simulink model "zerocross"  (Simulink 4.00)
settings: Solver=ode45  StartTime=0.0  StopTime=10.0  RelTol=1e-3
settings Model: LastModifiedBy=dev  LimitDataPoints=off  RTWOptions="-aExtMode=0 -aForceParamTrailComments=0 -aInlineInvariantSignals=0 -aLocalBlockOutputs=1 -aLogVarNameModifier=\"rt_\" -aRTWVerbose=1 -aRollThreshold=5 -aShowEliminatedStatements=1"  RTWInlineParameters=on  BlockReductionOpt=off

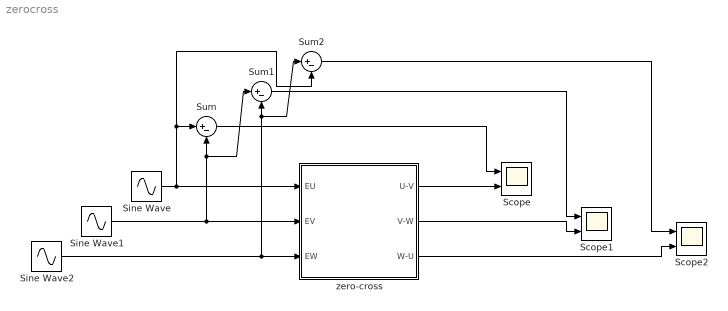
== system zerocross ==
  Scope : Scope  NumInputPorts=2
      settings: TimeRange=auto  YMin=-5~-5  YMax=5~5  SaveToWorkspace=off  SaveName=ScopeData  MaxDataPoints=5000
  Scope1 : Scope  NumInputPorts=2
      settings: TimeRange=auto  YMin=-5~-5  YMax=5~5  SaveToWorkspace=off  MaxDataPoints=5000
  Scope2 : Scope  NumInputPorts=2
      settings: TimeRange=auto  YMin=-5~-5  YMax=5~5  SaveToWorkspace=off  SaveName=ScopeData2  MaxDataPoints=5000
  Sine Wave : Sin  Amplitude=1  Frequency=10  Phase=0  SampleTime=0
  Sine Wave1 : Sin  Amplitude=1  Frequency=10  Phase=2*pi/3  SampleTime=0
  Sine Wave2 : Sin  Amplitude=1  Frequency=10  Phase=-2*pi/3  SampleTime=0
  Sum : Sum  Inputs=|+-  SaturateOnIntegerOverflow=on
  Sum1 : Sum  Inputs=|+-  SaturateOnIntegerOverflow=on
  Sum2 : Sum  Inputs=|+-  SaturateOnIntegerOverflow=on
  zero-cross : Subsystem
      settings: RTWFcnNameOpts=Auto  RTWFileNameOpts=Auto
      mask Description: The block detects the zero crossing of the inputs. For accurate results use the  rising edge only.
  wires:
  Sine Wave/1 -> zero-cross/1(EU), Sum/1, Sum2/2
  Sine Wave1/1 -> zero-cross/2(EV), Sum/2, Sum1/1
  Sine Wave2/1 -> zero-cross/3(EW), Sum1/2, Sum2/1
  zero-cross/1(U-V) -> Scope/2
  Sum/1 -> Scope/1
  Sum1/1 -> Scope1/1
  zero-cross/2(V-W) -> Scope1/2
  Sum2/1 -> Scope2/1
  zero-cross/3(W-U) -> Scope2/2

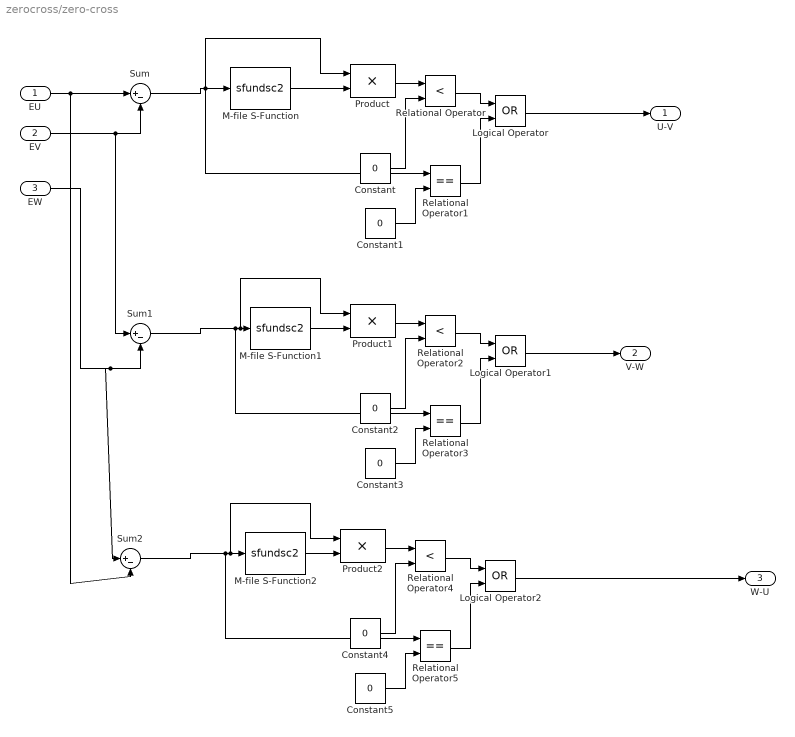
== system zerocross/zero-cross ==
  EU : Inport  Port=1
  EV : Inport  Port=2
  EW : Inport  Port=3
  Constant{,1..5} (6 alike) : Constant  Value=0
  Logical Operator : Logic  Operator=OR  Inputs=2
  Logical Operator1 : Logic  Operator=OR  Inputs=2
  Logical Operator2 : Logic  Operator=OR  Inputs=2
  M-file S-Function : S-Function  FunctionName=sfundsc2  PortCounts=[]  SFunctionModules=''
      mask Type: S-function: sfun_dsc2
      mask Description: This is a M-file S-function which demonstrates how toimplement an unit delay.
      mask Display: disp('Unit delay')
  M-file S-Function1 : S-Function  FunctionName=sfundsc2  PortCounts=[]  SFunctionModules=''
      mask Type: S-function: sfun_dsc2
      mask Description: This is a M-file S-function which demonstrates how toimplement an unit delay.
      mask Display: disp('Unit delay')
  M-file S-Function2 : S-Function  FunctionName=sfundsc2  PortCounts=[]  SFunctionModules=''
      mask Type: S-function: sfun_dsc2
      mask Description: This is a M-file S-function which demonstrates how toimplement an unit delay.
      mask Display: disp('Unit delay')
  Product : Product  Inputs=2  Multiplication=Element-wise(.*)  SaturateOnIntegerOverflow=on
  Product1 : Product  Inputs=2  Multiplication=Element-wise(.*)  SaturateOnIntegerOverflow=on
  Product2 : Product  Inputs=2  Multiplication=Element-wise(.*)  SaturateOnIntegerOverflow=on
  Relational Operator : RelationalOperator  Operator=<
  Relational Operator1 : RelationalOperator  Operator===
  Relational Operator2 : RelationalOperator  Operator=<
  Relational Operator3 : RelationalOperator  Operator===
  Relational Operator4 : RelationalOperator  Operator=<
  Relational Operator5 : RelationalOperator  Operator===
  Sum : Sum  Inputs=|+-  SaturateOnIntegerOverflow=on
  Sum1 : Sum  Inputs=|+-  SaturateOnIntegerOverflow=on
  Sum2 : Sum  Inputs=|+-  SaturateOnIntegerOverflow=on
  U-V : Outport  Port=1
  V-W : Outport  Port=2
  W-U : Outport  Port=3
  wires:
  Sum/1 -> Relational Operator1/1, Product/1, M-file S-Function/1
  M-file S-Function/1 -> Product/2
  Product/1 -> Relational Operator/1
  Constant/1 -> Relational Operator/2
  Constant1/1 -> Relational Operator1/2
  Relational Operator/1 -> Logical Operator/1
  Relational Operator1/1 -> Logical Operator/2
  Logical Operator/1 -> U-V/1
  EU/1 -> Sum/1, Sum2/2
  EV/1 -> Sum/2, Sum1/1
  Sum1/1 -> Relational Operator3/1, Product1/1, M-file S-Function1/1
  M-file S-Function1/1 -> Product1/2
  Product1/1 -> Relational Operator2/1
  Constant2/1 -> Relational Operator2/2
  Constant3/1 -> Relational Operator3/2
  Relational Operator2/1 -> Logical Operator1/1
  Relational Operator3/1 -> Logical Operator1/2
  Logical Operator1/1 -> V-W/1
  EW/1 -> Sum1/2, Sum2/1
  Sum2/1 -> M-file S-Function2/1, Product2/1, Relational Operator5/1
  M-file S-Function2/1 -> Product2/2
  Product2/1 -> Relational Operator4/1
  Constant4/1 -> Relational Operator4/2
  Constant5/1 -> Relational Operator5/2
  Relational Operator4/1 -> Logical Operator2/1
  Relational Operator5/1 -> Logical Operator2/2
  Logical Operator2/1 -> W-U/1
